simulink model "simul1_PID"  (R2022b)
settings: Solver=FixedStepAuto  StartTime=0.0  StopTime=20  FixedStep=0.001  RelTol=1e-3
undefined symbols (not defined in the file): awu, degs2rpm, der, drv, gbox, mot, National_Instruments, PCI, pid, real, rpm2degs, rpm2rads, sens, simul, Ts
libraries: simulink x4, sldrtlib x3
settings Model: SimulationMode=external  ExtModeTrigDuration=50001  ExtModeTrigDurationFloating=50001  Creator=perondavid  LastModifiedBy=david
settings DataIOCC: LoggingToFile=on
settings HardwareCC: ProdBitPerLong=64  ProdHWDeviceType=Intel->x86-64 (Linux 64)
settings RTWCC: Description=Simulink Desktop Real-Time  SystemTargetFile=sldrt.tlc  TemplateMakefile=sldrt.tmf  RTWCompilerOptimization=on
settings CodeAppCC: MaxIdLength=95
settings SimulinkDesktopRealTimeCC: TargetLibSuffix=_sldrt.a  TargetPreCompLibLocation=C:\Program Files\MATLAB\R2022b\toolbox\sldrt\lib\win64

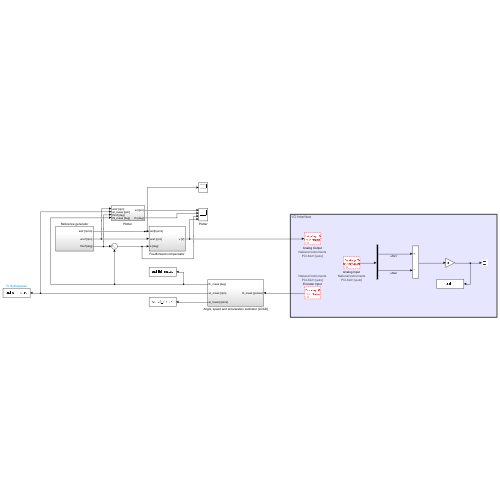
[thumbnail: Simulink's stored preview of the top-level diagram]
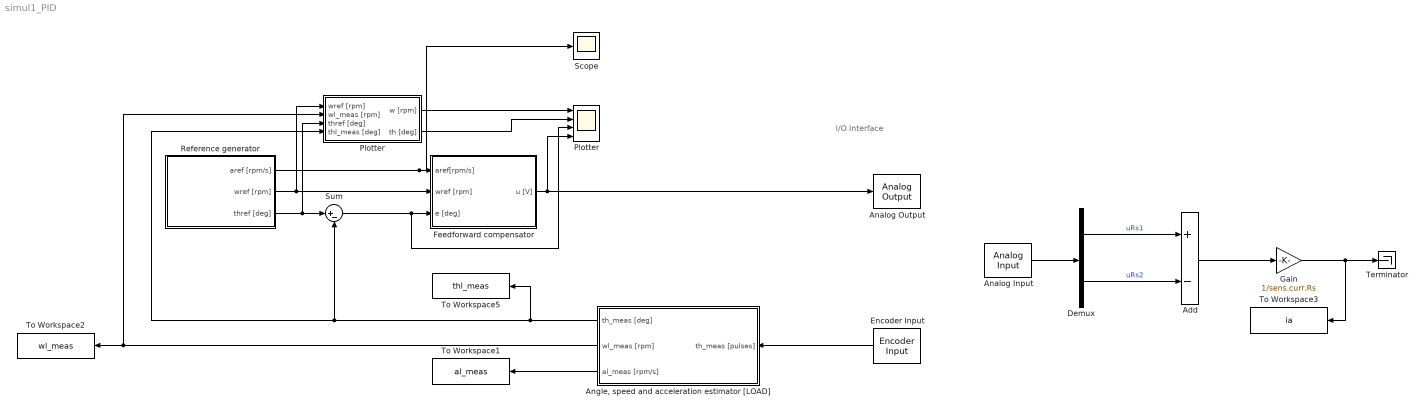
== system simul1_PID ==
  note: I/O Interface
  Add : Sum  Inputs=+-
  Analog Input : sldrtlib/Analog Input  SampleTime=-1  MaxMissedTicks=10  ShowMissedTicks=off  YieldWhenWaiting=off  DrvName=National_Instruments/PCI-6221  DrvAddress=4294967295  DrvOptions=[0 0 0 2 0]  Channels=[1, 2]  RangeMode=1  VoltRange=1  DataType=1
      settings: AttributesFormatString=National Instruments\nPCI-6221 [auto]
  Analog Output : sldrtlib/Analog Output  SampleTime=-1  MaxMissedTicks=10  ShowMissedTicks=off  YieldWhenWaiting=off  DrvName=National_Instruments/PCI-6221  DrvAddress=4294967295  DrvOptions=[0 0 0 2 0]  Channels=1  RangeMode=1  VoltRange=1  InitialValue=0  FinalValue=0
      settings: AttributesFormatString=National Instruments\nPCI-6221 [auto]
  "Angle, speed and acceleration estimator [LOAD]" : Subsystem
  Demux : Demux  Outputs=2
  Encoder Input : sldrtlib/Encoder Input  SampleTime=-1  MaxMissedTicks=10  ShowMissedTicks=off  YieldWhenWaiting=off  DrvName=National_Instruments/PCI-6221  DrvAddress=4294967295  DrvOptions=[0 0 0 2 0]  Channels=1  QuadMode=3  IndexPulse=1  InputFilter=Inf  DataType=1
      settings: AttributesFormatString=National Instruments\nPCI-6221 [auto]
  Feedforward compensator : Subsystem
  Gain : Gain  Gain=1/sens.curr.Rs
  Plotter : Scope  NumInputPorts=4
  "Plotter " : Subsystem
  Reference generator : Subsystem
  Scope : Scope
  Sum : Sum  Inputs=|+-
  Terminator : Terminator
  To Workspace1 : ToWorkspace  VariableName=al_meas  SaveFormat=Structure With Time  SampleTime=Ts
  To Workspace2 : ToWorkspace  VariableName=wl_meas  SaveFormat=Structure With Time  SampleTime=Ts
  To Workspace3 : ToWorkspace  VariableName=ia  SaveFormat=Structure With Time  SampleTime=Ts
  To Workspace5 : ToWorkspace  VariableName=thl_meas  SaveFormat=Structure With Time  SampleTime=Ts
  wires:
  Demux/1 -> Add/1  "uRs1"
  Demux/2 -> Add/2  "uRs2"
  Add/1 -> Gain/1
  Gain/1 -> To Workspace3/1, Terminator/1
  Analog Input/1 -> Demux/1
  Reference generator/1(aref [rpm/s]) -> Scope/1, Feedforward compensator/1(aref[rpm/s])
  Reference generator/3(thref [deg]) -> "Plotter "/3(thref [deg]), Sum/1
  "Angle, speed and acceleration estimator [LOAD]"/2(wl_meas [rpm]) -> To Workspace2/1, "Plotter "/2(wl_meas [rpm])
  "Plotter "/1(w [rpm]) -> Plotter/1
  "Plotter "/2(th [deg]) -> Plotter/2
  Feedforward compensator/1(u [V]) -> Analog Output/1, Plotter/4
  Sum/1 -> Plotter/3, Feedforward compensator/3(e [deg])
  Reference generator/2(wref [rpm]) -> "Plotter "/1(wref [rpm]), Feedforward compensator/2(wref [rpm])
  "Angle, speed and acceleration estimator [LOAD]"/3(al_meas [rpm/s]) -> To Workspace1/1
  "Angle, speed and acceleration estimator [LOAD]"/1(th_meas [deg]) -> "Plotter "/4(thl_meas [deg]), Sum/2, To Workspace5/1
  Encoder Input/1 -> "Angle, speed and acceleration estimator [LOAD]"/1(th_meas [pulses])

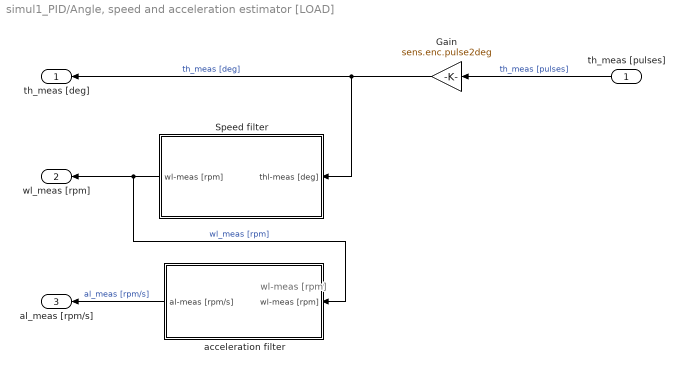
== system simul1_PID/Angle, speed and acceleration estimator [LOAD] ==
  note: wl-meas [rpm]
  th_meas [pulses] : Inport
  Gain : Gain  Gain=sens.enc.pulse2deg
  Speed filter : Subsystem
  acceleration filter : Subsystem
  th_meas [deg] : Outport
  wl_meas [rpm] : Outport  Port=2
  al_meas [rpm/s] : Outport  Port=3
  wires:
  Speed filter/1(wl-meas [rpm]) -> acceleration filter/1(wl-meas [rpm]), wl_meas [rpm]/1  "wl_meas [rpm]"
  th_meas [pulses]/1 -> Gain/1  "th_meas [pulses]"
  Gain/1 -> Speed filter/1(thl-meas [deg]), th_meas [deg]/1  "th_meas [deg]"
  acceleration filter/1(al-meas [rpm/s]) -> al_meas [rpm/s]/1  "al_meas [rpm/s]"

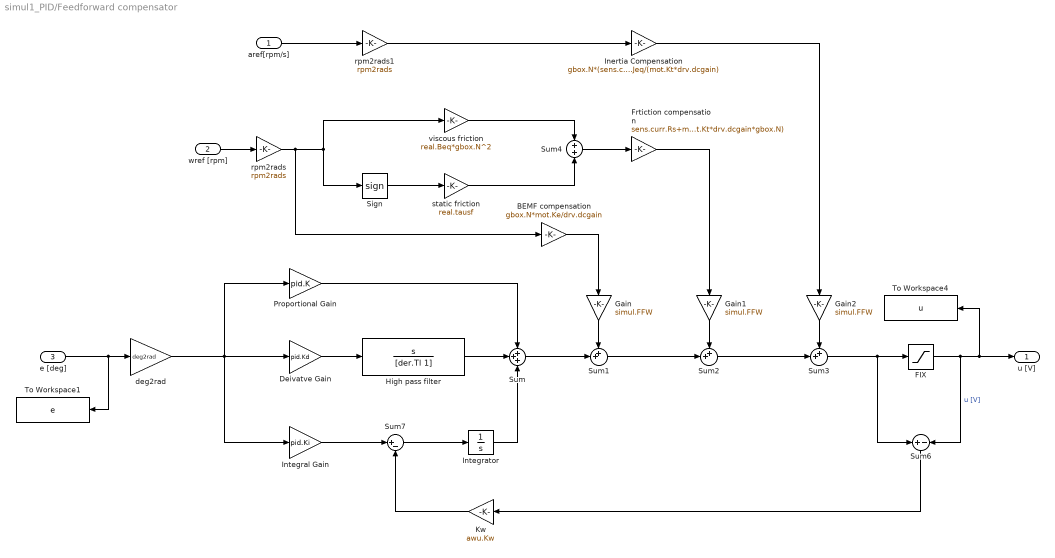
== system simul1_PID/Feedforward compensator ==
  aref[rpm/s] : Inport
  wref [rpm] : Inport  Port=2
  e [deg] : Inport  Port=3
  BEMF compensation : Gain  Gain=gbox.N*mot.Ke/drv.dcgain
  Deivatve Gain : Gain  Gain=pid.Kd
  "FIX " : Saturate  UpperLimit=10  LowerLimit=-10
  Frtiction compensation : Gain  Gain=sens.curr.Rs+mot.R/(mot.Kt*drv.dcgain*gbox.N)
  Gain : Gain  Gain=simul.FFW
  Gain1 : Gain  Gain=simul.FFW
  Gain2 : Gain  Gain=simul.FFW
  High pass filter : TransferFcn  Numerator=[1 0]  Denominator=[der.Tl 1]
  Inertia Compensation : Gain  Gain=gbox.N*(sens.curr.Rs+mot.R)*real.Jeq/(mot.Kt*drv.dcgain)
  Integral Gain : Gain  Gain=pid.Ki
  Integrator : Integrator
  Kw : Gain  Gain=awu.Kw
  Proportional Gain : Gain  Gain=pid.K
  Sign : Signum
  Sum : Sum  Inputs=+++
  Sum1 : Sum  Inputs=++|
  Sum2 : Sum  Inputs=++|
  Sum3 : Sum  Inputs=++|
  Sum4 : Sum
  Sum6 : Sum  Inputs=+-
  Sum7 : Sum  Inputs=|+-
  To Workspace1 : ToWorkspace  VariableName=e  SaveFormat=Structure With Time  SampleTime=Ts
  To Workspace4 : ToWorkspace  VariableName=u  SaveFormat=Structure With Time  SampleTime=Ts
  deg2rad : Gain  Gain=deg2rad
  rpm2rads : Gain  Gain=rpm2rads
  rpm2rads1 : Gain  Gain=rpm2rads
  static friction : Gain  Gain=real.tausf
  viscous friction : Gain  Gain=real.Beq*gbox.N^2
  u [V] : Outport
  wires:
  Sum2/1 -> Sum3/2
  Sum1/1 -> Sum2/2
  static friction/1 -> Sum4/2
  viscous friction/1 -> Sum4/1
  Sum4/1 -> Frtiction compensation/1
  Integrator/1 -> Sum/3
  Deivatve Gain/1 -> High pass filter/1
  Proportional Gain/1 -> Sum/1
  deg2rad/1 -> Integral Gain/1, Deivatve Gain/1, Proportional Gain/1
  High pass filter/1 -> Sum/2
  e [deg]/1 -> To Workspace1/1, deg2rad/1
  Sum3/1 -> Sum6/1, "FIX "/1
  "FIX "/1 -> Sum6/2, To Workspace4/1, u [V]/1  "u [V]"
  Sum/1 -> Sum1/2
  wref [rpm]/1 -> rpm2rads/1
  aref[rpm/s]/1 -> rpm2rads1/1
  Sign/1 -> static friction/1
  rpm2rads/1 -> BEMF compensation/1, Sign/1, viscous friction/1
  rpm2rads1/1 -> Inertia Compensation/1
  Gain1/1 -> Sum2/1
  Gain/1 -> Sum1/1
  Gain2/1 -> Sum3/1
  Inertia Compensation/1 -> Gain2/1
  Frtiction compensation/1 -> Gain1/1
  BEMF compensation/1 -> Gain/1
  Sum6/1 -> Kw/1
  Kw/1 -> Sum7/2
  Sum7/1 -> Integrator/1
  Integral Gain/1 -> Sum7/1

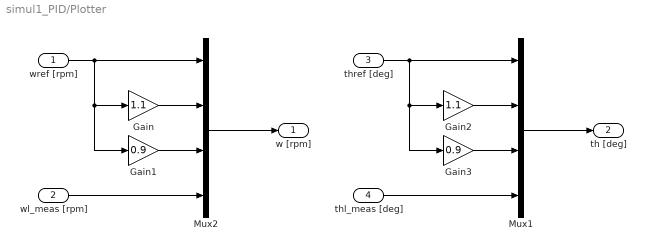
== system simul1_PID/Plotter  ==
  wref [rpm] : Inport
  wl_meas [rpm] : Inport  Port=2
  thref [deg] : Inport  Port=3
  thl_meas [deg] : Inport  Port=4
  Gain : Gain  Gain=1.1
  Gain1 : Gain  Gain=0.9
  Gain2 : Gain  Gain=1.1
  Gain3 : Gain  Gain=0.9
  Mux1 : Mux
  Mux2 : Mux
  w [rpm] : Outport
  th [deg] : Outport  Port=2
  wires:
  wref [rpm]/1 -> Gain1/1, Gain/1, Mux2/1
  Mux2/1 -> w [rpm]/1
  wl_meas [rpm]/1 -> Mux2/4
  Gain/1 -> Mux2/2
  Gain1/1 -> Mux2/3
  thref [deg]/1 -> Gain3/1, Gain2/1, Mux1/1
  thl_meas [deg]/1 -> Mux1/4
  Gain2/1 -> Mux1/2
  Gain3/1 -> Mux1/3
  Mux1/1 -> th [deg]/1

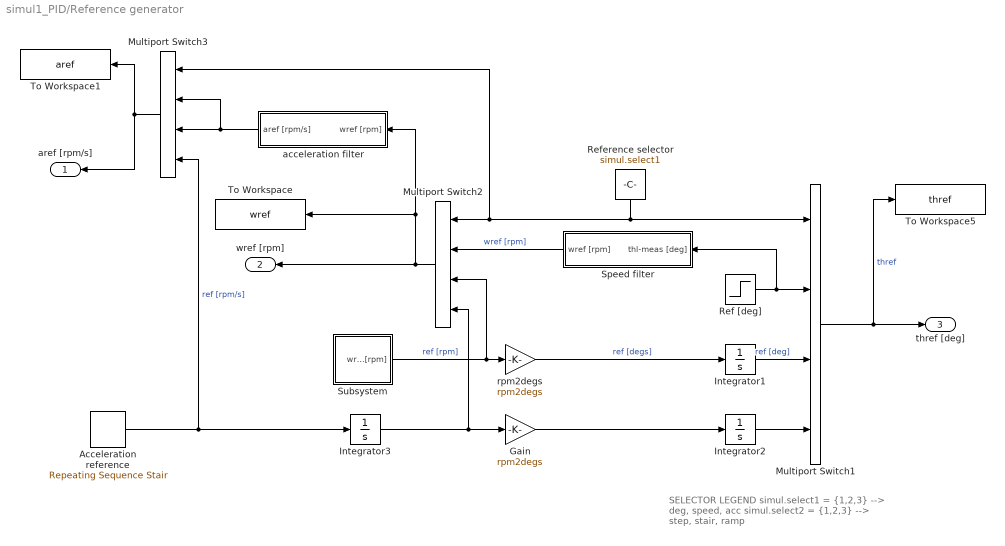
== system simul1_PID/Reference generator ==
  note: SELECTOR LEGEND
      |
      | simul.select1 = {1,2,3} --> deg, speed, acc
      | simul.select2 = {1,2,3} --> step, stair, ramp
  Acceleration reference : simulink/Sources/Repeating Sequence Stair  OutValues=[900 0 -900 -900 0 900].'  tsamp=0.5  OutMin=[]  OutMax=[]  OutDataTypeStr=double  OutputDataTypeScalingMode=double  OutDataType=fixdt(0,8)  ConRadixGroup=Best Precision: Vector-wise  OutScaling=2^-12
  Gain : Gain  Gain=rpm2degs
  Integrator1 : Integrator
  Integrator2 : Integrator
  Integrator3 : Integrator
  Multiport Switch1 : MultiPortSwitch  SaturateOnIntegerOverflow=off  InputSameDT=off
  Multiport Switch2 : MultiPortSwitch  SaturateOnIntegerOverflow=off  InputSameDT=off
  Multiport Switch3 : MultiPortSwitch  SaturateOnIntegerOverflow=off  InputSameDT=off
  Ref [deg] : Step  After=simul.stepdeg
  Reference selector : Constant  Value=simul.select1
  Speed filter : Subsystem
  Subsystem : Subsystem
  To Workspace : ToWorkspace  VariableName=wref  SaveFormat=Structure With Time  SampleTime=Ts
  To Workspace1 : ToWorkspace  VariableName=aref  SaveFormat=Structure With Time  SampleTime=Ts
  To Workspace5 : ToWorkspace  VariableName=thref  SaveFormat=Structure With Time  SampleTime=Ts
  acceleration filter : Subsystem
  rpm2degs : Gain  Gain=rpm2degs
  aref [rpm/s] : Outport
  wref [rpm] : Outport  Port=2
  thref [deg] : Outport  Port=3
  wires:
  Integrator1/1 -> Multiport Switch1/3  "ref [deg]"
  rpm2degs/1 -> Integrator1/1  "ref [degs]"
  Ref [deg]/1 -> Speed filter/1(thl-meas [deg]), Multiport Switch1/2
  Multiport Switch1/1 -> To Workspace5/1, thref [deg]/1  "thref"
  Subsystem/1(wref [rpm]) -> Multiport Switch2/3, rpm2degs/1  "ref [rpm]"
  Integrator2/1 -> Multiport Switch1/4
  Gain/1 -> Integrator2/1
  Integrator3/1 -> Multiport Switch2/4, Gain/1
  Acceleration reference/1 -> Integrator3/1, Multiport Switch3/4  "ref [rpm/s]"
  Multiport Switch2/1 -> wref [rpm]/1, To Workspace/1, acceleration filter/1(wref [rpm])
  Speed filter/1(wref [rpm]) -> Multiport Switch2/2  "wref [rpm]"
  Reference selector/1 -> Multiport Switch3/1, Multiport Switch2/1, Multiport Switch1/1
  acceleration filter/1(aref [rpm/s]) -> Multiport Switch3/3, Multiport Switch3/2
  Multiport Switch3/1 -> To Workspace1/1, aref [rpm/s]/1

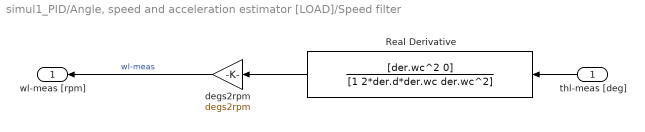
== system simul1_PID/Angle, speed and acceleration estimator [LOAD]/Speed filter ==
  thl-meas [deg] : Inport
  Real Derivative : TransferFcn  Numerator=[der.wc^2 0]  Denominator=[1 2*der.d*der.wc der.wc^2]
  degs2rpm : Gain  Gain=degs2rpm
  wl-meas [rpm] : Outport
  wires:
  thl-meas [deg]/1 -> Real Derivative/1
  degs2rpm/1 -> wl-meas [rpm]/1  "wl-meas"
  Real Derivative/1 -> degs2rpm/1

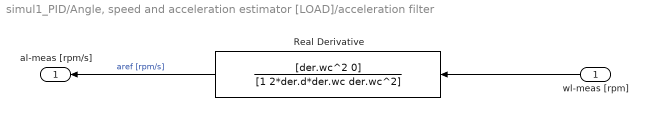
== system simul1_PID/Angle, speed and acceleration estimator [LOAD]/acceleration filter ==
  wl-meas [rpm] : Inport
  Real Derivative : TransferFcn  Numerator=[der.wc^2 0]  Denominator=[1 2*der.d*der.wc der.wc^2]
  al-meas [rpm/s] : Outport
  wires:
  wl-meas [rpm]/1 -> Real Derivative/1
  Real Derivative/1 -> al-meas [rpm/s]/1  "aref [rpm/s]"

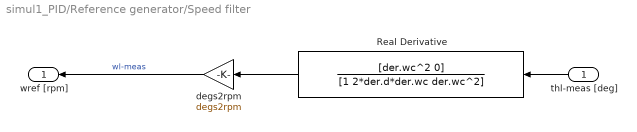
== system simul1_PID/Reference generator/Speed filter ==
  thl-meas [deg] : Inport
  Real Derivative : TransferFcn  Numerator=[der.wc^2 0]  Denominator=[1 2*der.d*der.wc der.wc^2]
  degs2rpm : Gain  Gain=degs2rpm
  wref [rpm] : Outport
  wires:
  thl-meas [deg]/1 -> Real Derivative/1
  degs2rpm/1 -> wref [rpm]/1  "wl-meas"
  Real Derivative/1 -> degs2rpm/1

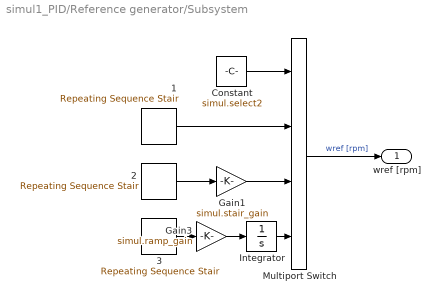
== system simul1_PID/Reference generator/Subsystem ==
  1 : simulink/Sources/Repeating Sequence Stair  OutValues=[250 -250].'  tsamp=1  OutMin=[]  OutMax=[]  OutDataTypeStr=double  OutputDataTypeScalingMode=double  OutDataType=fixdt(0,8)  ConRadixGroup=Best Precision: Vector-wise  OutScaling=2^-12
  2 : simulink/Sources/Repeating Sequence Stair  OutValues=[50 100 150 200 250 300 350 400 450 450].'  tsamp=5  OutMin=[]  OutMax=[]  OutDataTypeStr=double  OutputDataTypeScalingMode=double  OutDataType=fixdt(0,8)  ConRadixGroup=Best Precision: Vector-wise  OutScaling=2^-12
  3 : simulink/Sources/Repeating Sequence Stair  OutValues=[450 -450].'  tsamp=1  OutMin=[]  OutMax=[]  OutDataTypeStr=double  OutputDataTypeScalingMode=double  OutDataType=fixdt(0,8)  ConRadixGroup=Best Precision: Vector-wise  OutScaling=2^-12
  Constant : Constant  Value=simul.select2
  Gain1 : Gain  Gain=simul.stair_gain
  Gain3 : Gain  Gain=simul.ramp_gain
  Integrator : Integrator
  Multiport Switch : MultiPortSwitch  SaturateOnIntegerOverflow=off  InputSameDT=off
  wref [rpm] : Outport
  wires:
  1/1 -> Multiport Switch/2
  Gain3/1 -> Integrator/1
  Integrator/1 -> Multiport Switch/4
  Multiport Switch/1 -> wref [rpm]/1  "wref [rpm]"
  Gain1/1 -> Multiport Switch/3
  Constant/1 -> Multiport Switch/1
  3/1 -> Gain3/1
  2/1 -> Gain1/1

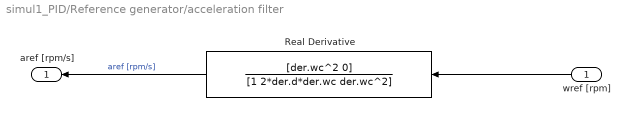
== system simul1_PID/Reference generator/acceleration filter ==
  wref [rpm] : Inport
  Real Derivative : TransferFcn  Numerator=[der.wc^2 0]  Denominator=[1 2*der.d*der.wc der.wc^2]
  aref [rpm/s] : Outport
  wires:
  wref [rpm]/1 -> Real Derivative/1
  Real Derivative/1 -> aref [rpm/s]/1  "aref [rpm/s]"
